simulink library "MyLib"  (Simulink 6.3)
InitFcn:
  | %% DSPBuilder Start
  | alt_dspbuilder_update_model(bdroot)
  | %% DSPBuilder End
libraries: allblocks_alteradspbuilder2 x1
settings Model: LastModifiedBy=gnixon  ExtModeAutoUpdateStatusClock=off  StrictBusMsg=None

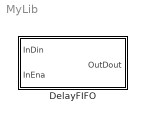
== system MyLib ==
  DelayFIFO : Subsystem  mask(SubSystem AlteraBlockSet){d=17}
      mask prompts: d "Delay"
      mask help:
      | RAM Based Delay Element
      |
      | Altera Corporation
      mask Display:
      | port_label('input',1,'din');
      | port_label('input',2,'ena');
      | port_label('output',1,'dout');
      | fprintf('Delay %d',d)

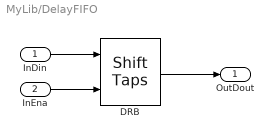
== system MyLib/DelayFIFO ==
  InDin : Inport
  InEna : Inport  Port=2
  DRB : allblocks_alteradspbuilder2/Shift Taps  number_of_taps=1  tap_distance=d  use_shiftout=off  use_ena=on  use_sclr=off  use_dedicated_circuitry=off  ram_type=AUTO
  OutDout : Outport
  wires:
  DRB/1 -> OutDout/1
  InEna/1 -> DRB/2
  InDin/1 -> DRB/1
